simulink model "rgbFilter_2025a"  (R2025a)
settings: Solver=FixedStepDiscrete  StartTime=0.0  StopTime=2  RelTol=1e-3
values from neighbouring files (symbols this model uses):
  blueMax = 255    [setup.m]
  greenMax = 255    [setup.m]
  redMax = 0    [setup.m]
undefined symbols (not defined in the file or in its folder): gray
libraries: hdlsllib x13, visionhdlio x3, visionsources x1
Description:
  | Sobel Edge Detection Using the MATLAB(R) Function Block
  | This example shows how to use HDL Coder(TM) to check,
  | generate, and verify HDL code for a Sobel Edge Detection
  | block built using the MATLAB Function block.
settings Model: FPTRunName=Active  Creator=The MathWorks, Inc.  LastModifiedBy=gpsiee
settings SolverCC: AlgebraicLoopSolver=TrustRegion
settings DataIOCC: LimitDataPoints=on  SaveFormat=Array  SignalLogging=off  ReturnWorkspaceOutputs=off
settings OptimizationCC: BlockReduction=off  ConditionallyExecuteInputs=off  DefaultParameterBehavior=Inlined  ExpressionDepthLimit=2147483647.0  InitFltsAndDblsToZero=on  EfficientMapNaN2IntZero=off  LifeSpan=inf
settings DebuggingCC: AlgebraicLoopMsg=error  SaveWithParameterizedLinksMsg=none  UnderspecifiedInitializationDetection=Classic  MergeDetectMultiDrivingBlocksExec=none  SignalResolutionControl=TryResolveAllWithWarning  MultiTaskDSMMsg=warning  MultiTaskCondExecSysMsg=none  SingleTaskRateTransMsg=error  IntegerOverflowMsg=none  ParameterPrecisionLossMsg=none  FcnCallInpInsideContextMsg=warning  UnconnectedInputMsg=warning  UnconnectedOutputMsg=warning  UnconnectedLineMsg=warning  AllowSymbolicDim=off  StateNameClashWarn=warning  StrictBusMsg=ErrorOnBusTreatedAsVector  SFUnexpectedBacktrackingDiag=warning  SFNoUnconditionalDefaultTransitionDiag=warning  SFExecutionAtInitializationDiag=none  IntegerSaturationMsg=none  ArithmeticOperatorsInVariantConditions=warning
settings HardwareCC: ProdBitPerPointer=32.0  ProdBitPerSizeT=32.0  ProdBitPerPtrDiffT=32.0  ProdLargestAtomicFloat=None  ProdIntDivRoundTo=Undefined  ProdEndianess=Unspecified  ProdWordSize=32.0  ProdHWDeviceType=ASIC/FPGA  TargetHWDeviceType=32-bit Generic  ProdEqTarget=off
settings ModelReferenceCC: EnableRefExpFcnMdlSchedulingChecks=on  PropagateSignalLabelsOutOfModel=off
settings SFSimCC: SimUseLocalCustomCode=off  CustomCodeUndefinedFunction=UseInterfaceOnly
settings RTWCC: RTWUseLocalCustomCode=off  GPUComputeCapability=3.5  DLArmComputeVersion=19.05
settings CodeAppCC: StateflowObjectComments=on
settings GRTTargetCC: TargetFcnLib=ansi_tfl_tmw.mat  TargetLangStandard=C89/C90 (ANSI)  CombineOutputUpdateFcns=off  GRTInterface=on
settings ConfigComp: CovMetricSettings=dw  CovSaveCumulativeToWorkspaceVar=on  CovSaveSingleToWorkspaceVar=on  CovExternalEMLEnable=off

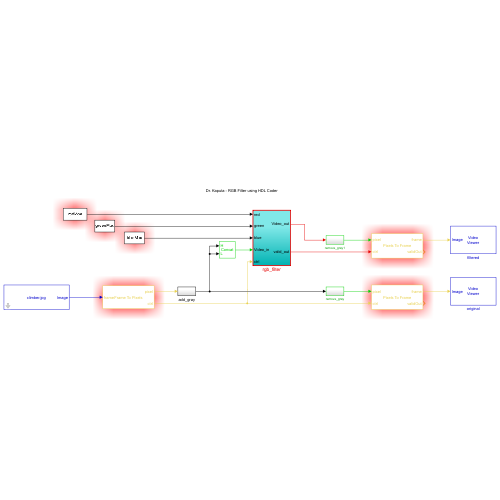
[thumbnail: Simulink's stored preview of the top-level diagram]
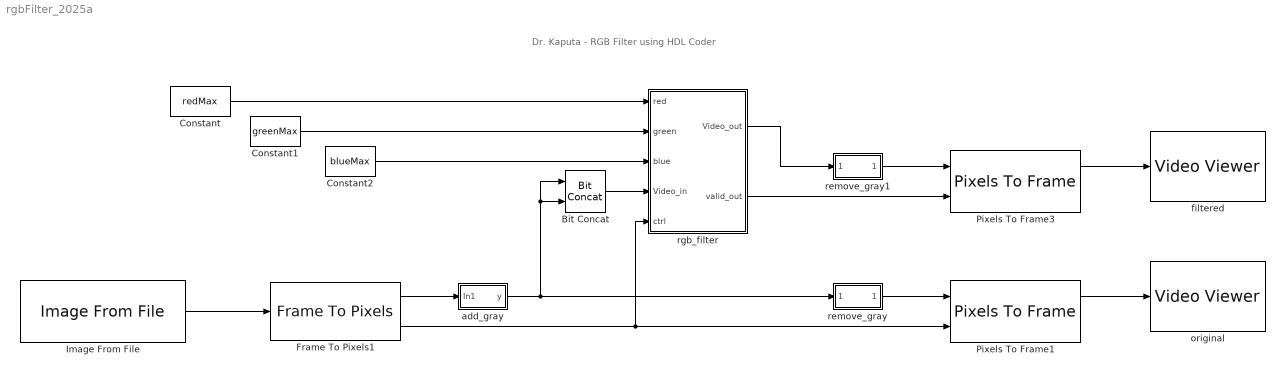
== system rgbFilter_2025a ==
  note: Dr. Kaputa - RGB Filter using HDL Coder
  Bit Concat : hdlsllib/Logic and Bit Operations/Bit Concat  numInputs=2
  Constant : Constant  Value=redMax  OutDataTypeStr=uint8  SampleTime=-1
  Constant1 : Constant  Value=greenMax  OutDataTypeStr=uint8  SampleTime=-1
  Constant2 : Constant  Value=blueMax  OutDataTypeStr=uint8  SampleTime=-1
  Frame To Pixels1 : visionhdlio/Frame To Pixels  NumComponents=3  NumPixels=1  VideoFormat=Custom  ActivePixelsPerLine=R  ActiveVideoLines=C  TotalPixelsPerLine=R  TotalVideoLines=C  StartingActiveLine=1  FrontPorch=0  SampleTime=0  VideoFormatCache=Custom  ActivePixelsPerLineCache=R  ActiveVideoLinesCache=C  TotalPixelsPerLineCache=R  TotalVideoLinesCache=C  StartingActiveLineCache=1  FrontPorchCache=0
  Image From File : visionsources/Image From File  Tag=vipblks_nd  FileName=climber.jpg  Ts=1  imagePorts=One multidimensional signal  OutPortLabels=R|G|B  ImageDataType=Inherit from input image  sdImageDataType=uint(8)  Signed=on  WordLength=16  FractionLengthMode=User-defined  FractionLength=15
  Pixels To Frame1 : visionhdlio/Pixels To Frame  NumComponents=3  NumPixels=1  VideoFormat=Custom  ActivePixelsPerLine=R  ActiveVideoLines=C  TotalPixelsPerLine=R  TotalVideoLines=C  VideoFormatCache=Custom  ActivePixelsPerLineCache=R  ActiveVideoLinesCache=C  TotalPixelsPerLineCache=R  TotalVideoLinesCache=C
  Pixels To Frame3 : visionhdlio/Pixels To Frame  NumComponents=3  NumPixels=1  VideoFormat=Custom  ActivePixelsPerLine=R  ActiveVideoLines=C  TotalPixelsPerLine=R  TotalVideoLines=C  VideoFormatCache=Custom  ActivePixelsPerLineCache=R  ActiveVideoLinesCache=C  TotalPixelsPerLineCache=R  TotalVideoLinesCache=C
  add_gray : Subsystem
  filtered : VideoViewer  colormapValue=gray(256)  FigPos=[320 850 1280 622.666666666667]
  original : VideoViewer  FigPos=[320 850 1280 623]
  remove_gray : Subsystem
  remove_gray1 : Subsystem
  rgb_filter : Subsystem  TreatAsAtomicUnit=on
  wires:
  Image From File/1 -> Frame To Pixels1/1
  Pixels To Frame1/1 -> original/1
  Frame To Pixels1/2 -> rgb_filter/5(ctrl), Pixels To Frame1/2
  remove_gray/1(RGBVector) -> Pixels To Frame1/1
  Frame To Pixels1/1 -> add_gray/1(In1)
  add_gray/1(y) -> Bit Concat/1, Bit Concat/2, remove_gray/1(RGB)
  Pixels To Frame3/1 -> filtered/1
  rgb_filter/1(Video_out) -> remove_gray1/1(RGB)
  rgb_filter/2(valid_out) -> Pixels To Frame3/2
  Bit Concat/1 -> rgb_filter/4(Video_in)
  remove_gray1/1(RGBVector) -> Pixels To Frame3/1
  Constant/1 -> rgb_filter/1(red)
  Constant1/1 -> rgb_filter/2(green)
  Constant2/1 -> rgb_filter/3(blue)

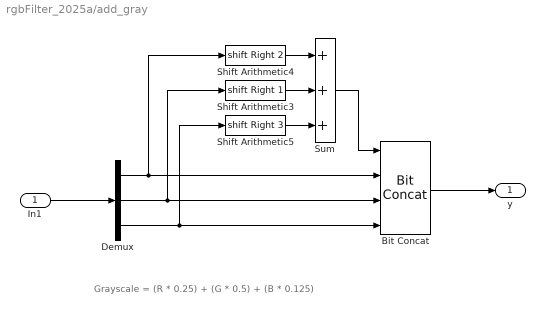
== system rgbFilter_2025a/add_gray ==
  note: Grayscale = (R * 0.25) + (G * 0.5) + (B * 0.125)
  In1 : Inport
  Bit Concat : hdlsllib/Logic and Bit Operations/Bit Concat  numInputs=4
  Demux : Demux  Outputs=3
  Shift Arithmetic3 : ArithShift  BitShiftNumber=1  BitShiftDirection=Right
  Shift Arithmetic4 : ArithShift  BitShiftNumber=2  BitShiftDirection=Right
  Shift Arithmetic5 : ArithShift  BitShiftNumber=3  BitShiftDirection=Right
  Sum : Sum  Inputs=+++  OutDataTypeStr=uint8
  y : Outport
  wires:
  Bit Concat/1 -> y/1
  In1/1 -> Demux/1
  Demux/2 -> Shift Arithmetic3/1, Bit Concat/3
  Demux/1 -> Shift Arithmetic4/1, Bit Concat/2
  Demux/3 -> Shift Arithmetic5/1, Bit Concat/4
  Sum/1 -> Bit Concat/1
  Shift Arithmetic4/1 -> Sum/1
  Shift Arithmetic3/1 -> Sum/2
  Shift Arithmetic5/1 -> Sum/3

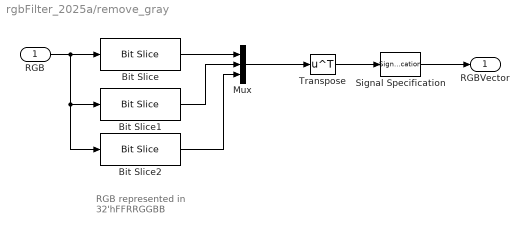
== system rgbFilter_2025a/remove_gray ==
  note: RGB represented in
      | 32'hFFRRGGBB
  RGB : Inport
  Bit Slice : hdlsllib/Logic and Bit Operations/Bit Slice  lidx=23  ridx=16
  Bit Slice1 : hdlsllib/Logic and Bit Operations/Bit Slice  lidx=15  ridx=8
  Bit Slice2 : hdlsllib/Logic and Bit Operations/Bit Slice  lidx=7  ridx=0
  Mux : Mux  Inputs=3
  Signal Specification : SignalSpecification
  Transpose : Math  Operator=transpose  SignedPower=on
  RGBVector : Outport  VectorParamsAs1DForOutWhenUnconnected=off
  wires:
  Signal Specification/1 -> RGBVector/1
  Transpose/1 -> Signal Specification/1
  RGB/1 -> Bit Slice/1, Bit Slice1/1, Bit Slice2/1
  Bit Slice1/1 -> Mux/2
  Bit Slice2/1 -> Mux/3
  Bit Slice/1 -> Mux/1
  Mux/1 -> Transpose/1

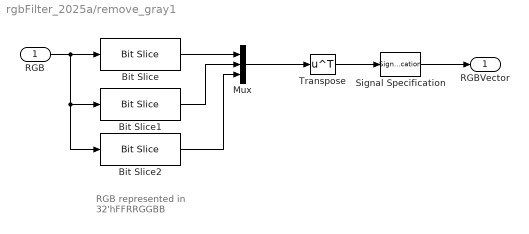
== system rgbFilter_2025a/remove_gray1 ==
  note: RGB represented in
      | 32'hFFRRGGBB
  RGB : Inport
  Bit Slice : hdlsllib/Logic and Bit Operations/Bit Slice  lidx=23  ridx=16
  Bit Slice1 : hdlsllib/Logic and Bit Operations/Bit Slice  lidx=15  ridx=8
  Bit Slice2 : hdlsllib/Logic and Bit Operations/Bit Slice  lidx=7  ridx=0
  Mux : Mux  Inputs=3
  Signal Specification : SignalSpecification
  Transpose : Math  Operator=transpose  SignedPower=on
  RGBVector : Outport  VectorParamsAs1DForOutWhenUnconnected=off
  wires:
  Signal Specification/1 -> RGBVector/1
  Transpose/1 -> Signal Specification/1
  RGB/1 -> Bit Slice/1, Bit Slice1/1, Bit Slice2/1
  Bit Slice1/1 -> Mux/2
  Bit Slice2/1 -> Mux/3
  Bit Slice/1 -> Mux/1
  Mux/1 -> Transpose/1

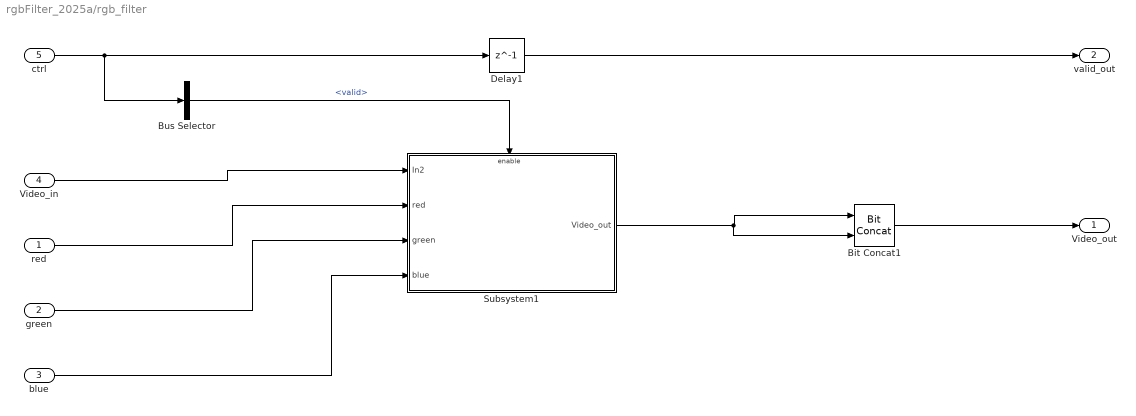
== system rgbFilter_2025a/rgb_filter ==
  red : Inport
  green : Inport  Port=2
  blue : Inport  Port=3
  Video_in : Inport  Port=4
  ctrl : Inport  Port=5
  Bit Concat1 : hdlsllib/Logic and Bit Operations/Bit Concat  numInputs=2
  Bus Selector : BusSelector  OutputSignals=valid
  Delay1 : Delay  DelayLength=1  InitialCondition=0
  Subsystem1 : Subsystem
  Video_out : Outport  VectorParamsAs1DForOutWhenUnconnected=off
  valid_out : Outport  Port=2  VectorParamsAs1DForOutWhenUnconnected=off
  wires:
  Video_in/1 -> Subsystem1/1(In2)
  ctrl/1 -> Bus Selector/1, Delay1/1
  Bus Selector/1 -> Subsystem1/Enable  "<valid>"
  red/1 -> Subsystem1/2(red)
  Delay1/1 -> valid_out/1
  green/1 -> Subsystem1/3(green)
  blue/1 -> Subsystem1/4(blue)
  Bit Concat1/1 -> Video_out/1
  Subsystem1/1(Video_out) -> Bit Concat1/2, Bit Concat1/1

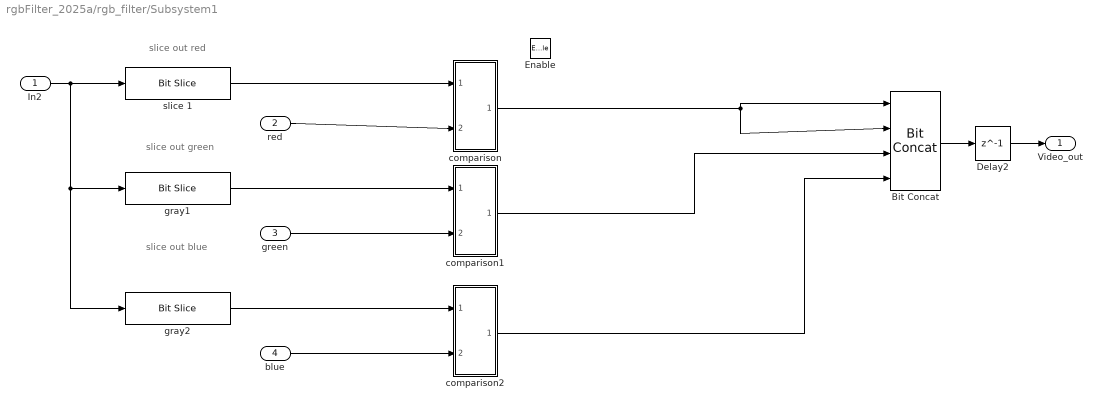
== system rgbFilter_2025a/rgb_filter/Subsystem1 ==
  note: slice out red
  note: slice out green
  note: slice out blue
  In2 : Inport
  red : Inport  Port=2
  green : Inport  Port=3
  blue : Inport  Port=4
  Enable : EnablePort
  Bit Concat : hdlsllib/Logic and Bit Operations/Bit Concat  numInputs=4
  Delay2 : Delay  DelayLength=1  InitialCondition=0
  comparison : Subsystem
  comparison1 : Subsystem
  comparison2 : Subsystem
  gray1 : hdlsllib/Logic and Bit Operations/Bit Slice  lidx=15  ridx=8
  gray2 : hdlsllib/Logic and Bit Operations/Bit Slice  lidx=7  ridx=0
  slice 1 : hdlsllib/Logic and Bit Operations/Bit Slice  lidx=23  ridx=16
  Video_out : Outport  InitialOutput=[0]
  wires:
  In2/1 -> gray1/1, gray2/1, slice 1/1
  Bit Concat/1 -> Delay2/1
  Delay2/1 -> Video_out/1
  gray1/1 -> comparison1/1(In1)
  gray2/1 -> comparison2/1(In1)
  comparison/1(Out1) -> Bit Concat/2, Bit Concat/1
  slice 1/1 -> comparison/1(In1)
  red/1 -> comparison/2(In2)
  green/1 -> comparison1/2(In2)
  blue/1 -> comparison2/2(In2)
  comparison1/1(Out1) -> Bit Concat/3
  comparison2/1(Out1) -> Bit Concat/4

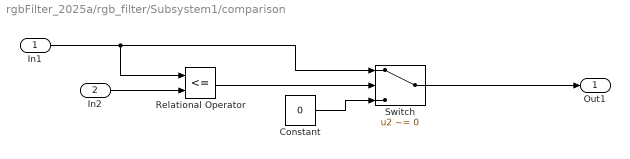
== system rgbFilter_2025a/rgb_filter/Subsystem1/comparison ==
  In1 : Inport
  In2 : Inport  Port=2
  Constant : Constant  Value=0  OutDataTypeStr=uint8  SampleTime=-1
  Relational Operator : RelationalOperator  Operator=<=  OutDataTypeStr=boolean  RndMeth=Simplest  InputSameDT=off
  Switch : Switch  Criteria=u2 ~= 0  SaturateOnIntegerOverflow=off  InputSameDT=off
  Out1 : Outport
  wires:
  Constant/1 -> Switch/3
  In1/1 -> Switch/1, Relational Operator/1
  Relational Operator/1 -> Switch/2
  In2/1 -> Relational Operator/2
  Switch/1 -> Out1/1

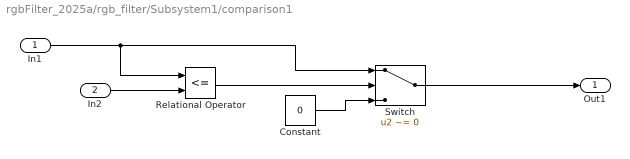
== system rgbFilter_2025a/rgb_filter/Subsystem1/comparison1 ==
  In1 : Inport
  In2 : Inport  Port=2
  Constant : Constant  Value=0  OutDataTypeStr=uint8  SampleTime=-1
  Relational Operator : RelationalOperator  Operator=<=  OutDataTypeStr=boolean  RndMeth=Simplest  InputSameDT=off
  Switch : Switch  Criteria=u2 ~= 0  SaturateOnIntegerOverflow=off  InputSameDT=off
  Out1 : Outport
  wires:
  Constant/1 -> Switch/3
  In1/1 -> Switch/1, Relational Operator/1
  Relational Operator/1 -> Switch/2
  In2/1 -> Relational Operator/2
  Switch/1 -> Out1/1

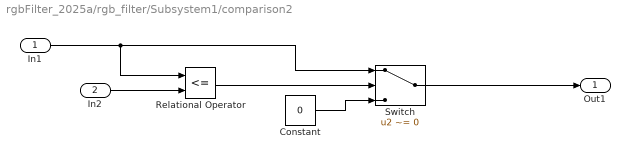
== system rgbFilter_2025a/rgb_filter/Subsystem1/comparison2 ==
  In1 : Inport
  In2 : Inport  Port=2
  Constant : Constant  Value=0  OutDataTypeStr=uint8  SampleTime=-1
  Relational Operator : RelationalOperator  Operator=<=  OutDataTypeStr=boolean  RndMeth=Simplest  InputSameDT=off
  Switch : Switch  Criteria=u2 ~= 0  SaturateOnIntegerOverflow=off  InputSameDT=off
  Out1 : Outport
  wires:
  Constant/1 -> Switch/3
  In1/1 -> Switch/1, Relational Operator/1
  Relational Operator/1 -> Switch/2
  In2/1 -> Relational Operator/2
  Switch/1 -> Out1/1
